simulink model "fl_blocks_2014a"  (R2014a)
settings: Solver=ode4  SolverMode=SingleTasking  StartTime=0.0  StopTime=tfin  FixedStep=0.1  RelTol=1e-3
values from neighbouring files (symbols this model uses):
  ga = i+2    [io_fl.m]
undefined symbols (not defined in the file or in its folder): mu_chua, ref_chua, u_chua
settings Model: CovMetricSettings=dwe  CovHtmlReporting=off  covSaveCumulativeToWorkspaceVar=off  CovSaveSingleToWorkspaceVar=off  CovExternalEMLEnable=on  CovSFcnEnable=on  Creator=carlonovara  LastModifiedBy=carlonovara
settings DataIOCC: LimitDataPoints=off  SaveFormat=StructureWithTime
settings DebuggingCC: MergeDetectMultiDrivingBlocksExec=error  SolverPrmCheckMsg=none  FrameProcessingCompatibilityMsg=error  SFUnexpectedBacktrackingDiag=error  SFNoUnconditionalDefaultTransitionDiag=error
settings HardwareCC: ProdBitPerPointer=64  ProdLargestAtomicFloat=Float  ProdIntDivRoundTo=Zero  ProdEndianess=LittleEndian  ProdHWDeviceType=Specified
settings ModelReferenceCC: PropagateSignalLabelsOutOfModel=on
settings GRTTargetCC: TargetLangStandard=C99 (ISO)  GeneratePreprocessorConditionals=Use local settings

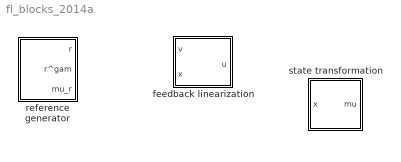
== system fl_blocks_2014a ==
  feedback linearization : Subsystem
  reference generator : Subsystem
  state transformation : Subsystem

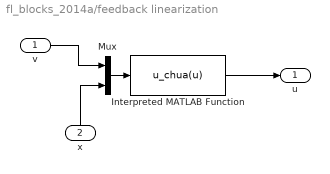
== system fl_blocks_2014a/feedback linearization ==
  v : Inport
  x : Inport  Port=2
  Interpreted MATLAB Function : MATLABFcn  MATLABFcn=u_chua(u)
  Mux : Mux  Inputs=2
  u : Outport
  wires:
  x/1 -> Mux/2
  Mux/1 -> Interpreted MATLAB Function/1
  v/1 -> Mux/1
  Interpreted MATLAB Function/1 -> u/1

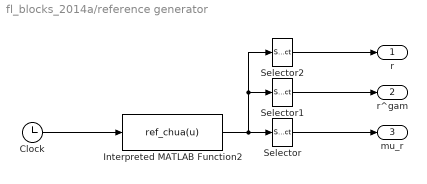
== system fl_blocks_2014a/reference generator ==
  Clock : Clock
  Interpreted MATLAB Function2 : MATLABFcn  MATLABFcn=ref_chua(u)
  Selector : Selector  InputPortWidth=ga+1  IndexOptions=Index vector (dialog)  Indices=1:ga  OutputSizes=1
  Selector1 : Selector  InputPortWidth=ga+1  IndexOptions=Index vector (dialog)  Indices=ga+1  OutputSizes=1
  Selector2 : Selector  InputPortWidth=ga+1  IndexOptions=Index vector (dialog)  Indices=1  OutputSizes=1
  r : Outport
  r^gam : Outport  Port=2
  mu_r : Outport  Port=3
  wires:
  Clock/1 -> Interpreted MATLAB Function2/1
  Selector1/1 -> r^gam/1
  Selector2/1 -> r/1
  Interpreted MATLAB Function2/1 -> Selector2/1, Selector1/1, Selector/1
  Selector/1 -> mu_r/1

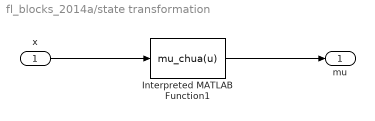
== system fl_blocks_2014a/state transformation ==
  x : Inport
  Interpreted MATLAB Function1 : MATLABFcn  MATLABFcn=mu_chua(u)
  mu : Outport
  wires:
  x/1 -> Interpreted MATLAB Function1/1
  Interpreted MATLAB Function1/1 -> mu/1
